simulink model "part1"  (R2017b)
settings: Solver=VariableStepAuto  StartTime=0.0  StopTime=0.5  MaxStep=0.000001  RelTol=1e-3
settings Model: Creator=ras19  LastModifiedBy=drone
settings CodeAppCC: StateflowObjectComments=on

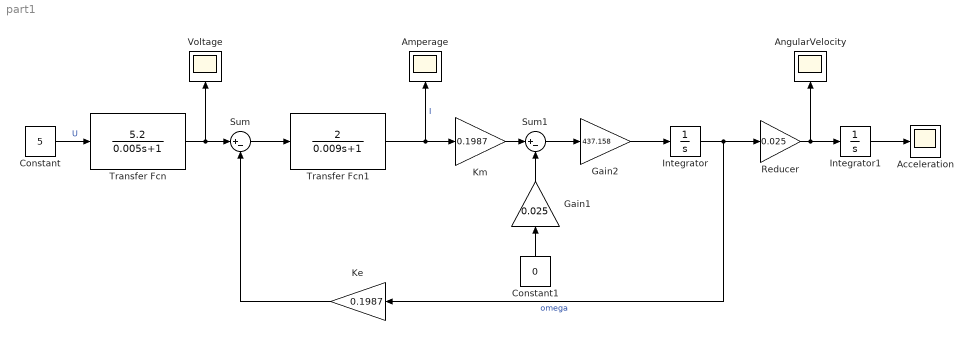
== system part1 ==
  Acceleration : Scope
  Amperage : Scope
  AngularVelocity : Scope
  Constant : Constant  Value=5
  Constant1 : Constant  Value=0
  Gain1 : Gain  Gain=0.025
  Gain2 : Gain  Gain=437.158
  Integrator : Integrator
  Integrator1 : Integrator
  Ke : Gain  Gain=0.1987
  Km : Gain  Gain=0.1987
  Reducer : Gain  Gain=0.025
  Sum : Sum  Inputs=|+-
  Sum1 : Sum  Inputs=|+-
  Transfer Fcn : TransferFcn  Numerator=[5.2]  Denominator=[0.005 1]
  Transfer Fcn1 : TransferFcn  Numerator=[2]  Denominator=[0.009 1]
  Voltage : Scope
  wires:
  Constant/1 -> Transfer Fcn/1  "U"
  Sum/1 -> Transfer Fcn1/1
  Transfer Fcn1/1 -> Km/1, Amperage/1  "I"
  Km/1 -> Sum1/1
  Constant1/1 -> Gain1/1
  Gain1/1 -> Sum1/2
  Sum1/1 -> Gain2/1
  Gain2/1 -> Integrator/1
  Ke/1 -> Sum/2
  Transfer Fcn/1 -> Sum/1, Voltage/1
  Reducer/1 -> AngularVelocity/1, Integrator1/1
  Integrator/1 -> Ke/1, Reducer/1  "omega"
  Integrator1/1 -> Acceleration/1
